simulink model "motor_nl21"  (R2021a)
settings: Solver=ode45  StartTime=0.0  StopTime=20  MaxStep=1e-3  RelTol=1e-3
values from neighbouring files (symbols this model uses):
  AL = double(subs(A_par))    [modeloMatematico.m]    (also in motor copy.m = double(subs(A,{x1,x2,x3,Vin,R,L,Ki,Kv,Jm,Jl,Bm,Bl,n,g,d,m},{; motor.m = double(subs(A,{x1,x2,x3,Vin,R,L,Ki,Kv,Jm,Jl,Bm,Bl,n,g,d,m},{; untitled.m = double(subs(A,{x1,x2,x3,u,M,g,R,L},{x10n,x20n,x30n,u0n,Mo,go)
  BL = double(subs(B_par))    [modeloMatematico.m]    (also in motor copy.m = double(subs(B,{x1,x2,x3,Vin,R,L,Ki,Kv,Jm,Jl,Bm,Bl,n,g,d,m},{; motor.m = double(subs(B,{x1,x2,x3,Vin,R,L,Ki,Kv,Jm,Jl,Bm,Bl,n,g,d,m},{; untitled.m = double(subs(B,{x1,x2,x3,u,M,g,R,L},{x10n,x20n,x30n,u0n,Mo,go)
  Bl0 = 0.0647    [modeloMatematico.m]    (also in motor copy.m = 0.147; motor.m = 0.05)
  Bm0 = 5.873e-9    (= 5.873e-09)    [modeloMatematico.m]    (also in motor copy.m = 5.862e-09; motor.m = 0.2)
  CL = double(subs(C_par))    [modeloMatematico.m]    (also in motor copy.m = [0 0 1/n0]; motor.m = [0 0 1/n0]; untitled.m = double(subs(C,{x1,x2,x3,u,M,g,R,L},{x10n,x20n,x30n,u0n,Mo,go)
  d0 = 0.065    [modeloMatematico.m]    (also in motor copy.m = 0.06587; motor.m = 0.1)
  DL = double(subs(D))    [modeloMatematico.m]    (also in motor copy.m = [0]; motor.m = [0]; untitled.m = double(subs(D,{x1,x2,x3,u,M,g,R,L},{x10n,x20n,x30n,u0n,Mo,go)
  g0 = 9.81    [modeloMatematico.m]    (also in motor copy.m; motor.m)
  GL = sysd.a    [untitled.m]
  HL = sysd.b    [untitled.m]
  Jl0 = 0.00000220756    (= 2.20756e-06)    [modeloMatematico.m]    (also in motor copy.m = 0.154364; motor.m = 0.02)
  Jm0 = 7.83568e-12    [modeloMatematico.m]    (also in motor copy.m = 7.83067e-12; motor.m = 0.01)
  Ki0 = 0.005119    [modeloMatematico.m]    (also in motor copy.m = 0.005012; motor.m = 2.3)
  Kv0 = 0.005119    [modeloMatematico.m]    (also in motor copy.m = 3.212e-11; motor.m = 1.5)
  L0 = 0.0013    [modeloMatematico.m]    (also in motor copy.m = 0.00051; motor.m = 0.04)
  m0 = 0.17244    [modeloMatematico.m]    (also in motor copy.m = 0.1045; motor.m = 0.1)
  n0 = 120    [modeloMatematico.m]    (also in motor copy.m; motor.m)
  R0 = 3.4    [modeloMatematico.m]    (also in motor copy.m = 3.9654; motor.m = 10)
  Tm = 2*pi/ws    (= 0.12036753462)    [motor copy.m]    (also in untitled.m = 0.01)
  Vin0 = R0*x10    [modeloMatematico.m]    (also in motor copy.m; motor.m = R*x10)
  x10 = (m0*g0*d0*sin(x30))/Ki0    [modeloMatematico.m]    (also in motor copy.m = (m0*g0*d0*sin(x30/n0))/Ki0; motor.m = (m*g*d*sin(x30/n0))/Ki0)
  x20 = 0    [modeloMatematico.m]    (also in motor copy.m; motor.m; untitled.m)
  x30 = thetaL0    (= 0)    [modeloMatematico.m]    (also in motor copy.m; motor.m; untitled.m = sqrt(M*g*x10))
settings Model: Creator=salones
settings DebuggingCC: UnconnectedInputMsg=none  UnconnectedOutputMsg=none  UnconnectedLineMsg=none
settings ModelReferenceCC: EnableRefExpFcnMdlSchedulingChecks=off
settings RTWCC: Description=Generic Real-Time Target  DLArmComputeVersion=20.02.1

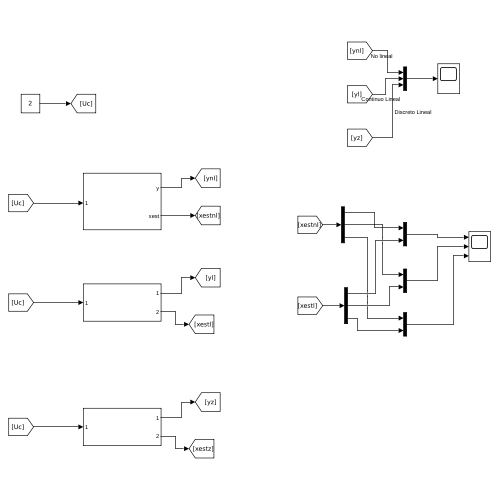
[thumbnail: Simulink's stored preview of the top-level diagram]
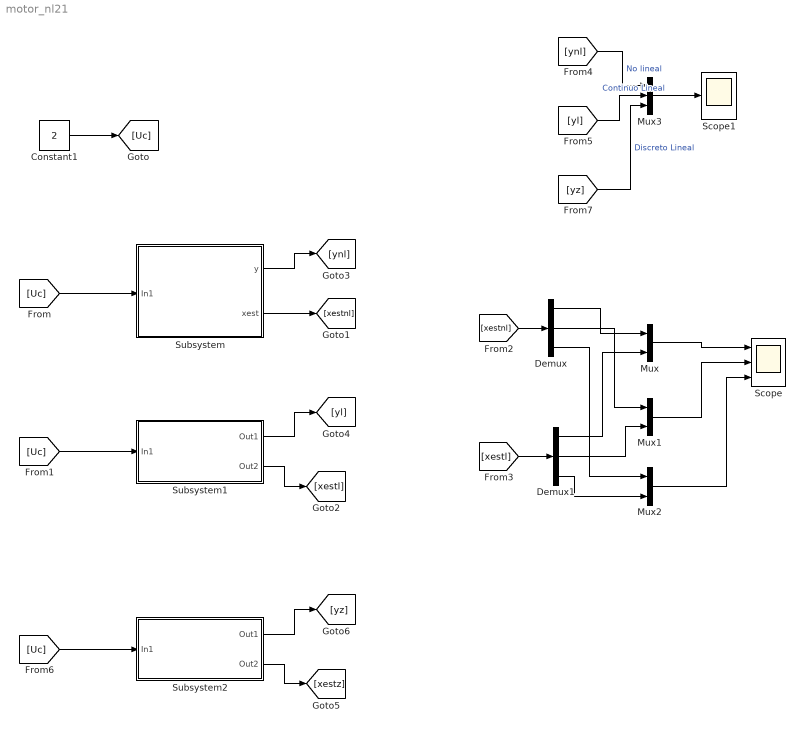
== system motor_nl21 ==
  Constant1 : Constant  Value=2
  Demux : Demux  Outputs=3
  Demux1 : Demux  Outputs=3
  Mux : Mux  Inputs=2
  Mux1 : Mux  Inputs=2
  Mux2 : Mux  Inputs=2
  Mux3 : Mux  Inputs=3
  Scope : Scope  NumInputPorts=3
  Scope1 : Scope
  Subsystem : Subsystem
  Subsystem1 : Subsystem
  Subsystem2 : Subsystem
  wires:
  Demux/1 -> Mux/1
  Demux1/1 -> Mux/2
  Mux/1 -> Scope/1
  Demux/2 -> Mux1/1
  Demux1/2 -> Mux1/2
  Demux/3 -> Mux2/1
  Demux1/3 -> Mux2/2
  Mux1/1 -> Scope/2
  Mux2/1 -> Scope/3
  Constant1/1 -> [Uc]
  [Uc] -> Subsystem/1(In1)
  [Uc] -> Subsystem1/1(In1)
  [xestnl] -> Demux/1
  [xestl] -> Demux1/1
  Subsystem/2(xest) -> [xestnl]
  Subsystem/1(y) -> [ynl]
  Subsystem1/1(Out1) -> [yl]
  Subsystem1/2(Out2) -> [xestl]
  Mux3/1 -> Scope1/1
  [ynl] -> Mux3/1  "No lineal"
  [yl] -> Mux3/2  "Continuo Lineal"
  Subsystem2/1(Out1) -> [yz]
  [Uc] -> Subsystem2/1(In1)
  Subsystem2/2(Out2) -> [xestz]
  [yz] -> Mux3/3  "Discreto Lineal"

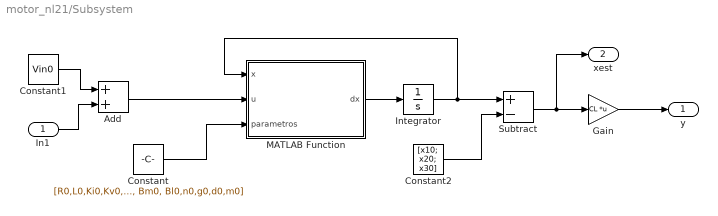
== system motor_nl21/Subsystem ==
  In1 : Inport
  Add : Sum
  Constant : Constant  Value=[R0,L0,Ki0,Kv0,Jm0, Jl0, Bm0, Bl0,n0,g0,d0,m0]
  Constant1 : Constant  Value=Vin0
  Constant2 : Constant  Value=[x10; x20; x30]
  Gain : Gain  Gain=CL  Multiplication=Matrix(K*u)
  Integrator : Integrator  InitialCondition=[x10; x20; x30]
  MATLAB Function : MATLAB Function  TreatAsAtomicUnit=on
  Subtract : Sum  Inputs=+-
  y : Outport
  xest : Outport  Port=2
  wires:
  Integrator/1 -> Subtract/1, MATLAB Function/1(x)
  Constant/1 -> MATLAB Function/3(parametros)
  In1/1 -> Add/2
  Constant1/1 -> Add/1
  Constant2/1 -> Subtract/2
  MATLAB Function/1(dx) -> Integrator/1
  Add/1 -> MATLAB Function/2(u)
  Subtract/1 -> xest/1, Gain/1
  Gain/1 -> y/1

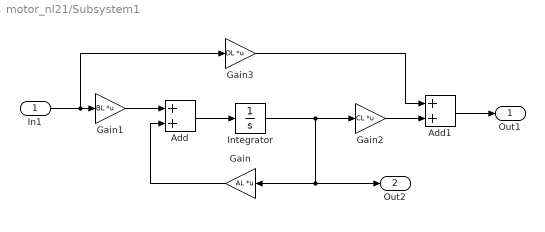
== system motor_nl21/Subsystem1 ==
  In1 : Inport
  Add : Sum
  Add1 : Sum
  Gain : Gain  Gain=AL  Multiplication=Matrix(K*u)
  Gain1 : Gain  Gain=BL  Multiplication=Matrix(K*u)
  Gain2 : Gain  Gain=CL  Multiplication=Matrix(K*u)
  Gain3 : Gain  Gain=DL  Multiplication=Matrix(K*u)
  Integrator : Integrator
  Out1 : Outport
  Out2 : Outport  Port=2
  wires:
  Integrator/1 -> Gain2/1, Gain/1, Out2/1
  Gain3/1 -> Add1/1
  Add/1 -> Integrator/1
  Gain1/1 -> Add/1
  Add1/1 -> Out1/1
  Gain/1 -> Add/2
  Gain2/1 -> Add1/2
  In1/1 -> Gain3/1, Gain1/1

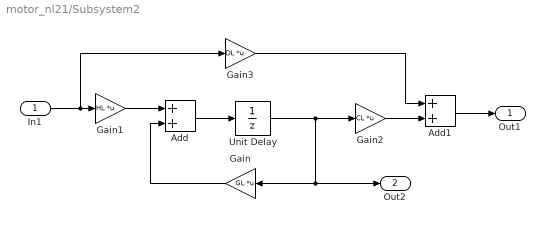
== system motor_nl21/Subsystem2 ==
  In1 : Inport
  Add : Sum
  Add1 : Sum
  Gain : Gain  Gain=GL  Multiplication=Matrix(K*u)
  Gain1 : Gain  Gain=HL  Multiplication=Matrix(K*u)
  Gain2 : Gain  Gain=CL  Multiplication=Matrix(K*u)
  Gain3 : Gain  Gain=DL  Multiplication=Matrix(K*u)
  Unit Delay : UnitDelay  SampleTime=Tm  HasFrameUpgradeWarning=on
  Out1 : Outport
  Out2 : Outport  Port=2
  wires:
  Unit Delay/1 -> Gain2/1, Gain/1, Out2/1
  Gain3/1 -> Add1/1
  Add/1 -> Unit Delay/1
  Gain1/1 -> Add/1
  Add1/1 -> Out1/1
  Gain/1 -> Add/2
  Gain2/1 -> Add1/2
  In1/1 -> Gain3/1, Gain1/1

== matlab function motor_nl21/Subsystem/MATLAB Function ==
  data: x input; u input; dx output; parametros input
function dx = fcn(x,u,parametros)

x1 = x(1);
x2 = x(2);
x3 = x(3);
Vin = u;

R = parametros(1);
L = parametros(2);
Ki = parametros(3);
Kv = parametros(4);
Jm = parametros(5);
Jl = parametros(6);
Bm = parametros(7);
Bl = parametros(8);
n = parametros(9);
g = parametros(10);
d = parametros(11);
m = parametros(12);

Jt = Jm + Jl/n;
f1 = (1/L)*(Vin - R*x1 - Kv*x2);
f2 = (1/Jt)*(Ki*x1 - (Bm + Bl/n)*x2 - m*g*d*sin(x3/n));
f3 = x2;
dx = [f1; f2; f3];
